simulink model "R7014E_QuadTankSim_IMC"  (R2025b)
settings: Solver=ode4  StartTime=0.0  StopTime=4000  FixedStep=0.01  RelTol=1e-3  EnableMultiTasking=on
values from neighbouring files (symbols this model uses):
  A1 = 28    [matlab_workspace.mat]
  a1 = 0.071    [matlab_workspace.mat]
  A2 = 32    [matlab_workspace.mat]
  a2 = 0.057    [matlab_workspace.mat]
  A3 = 28    [matlab_workspace.mat]
  a3 = 0.071    [matlab_workspace.mat]
  A4 = 32    [matlab_workspace.mat]
  a4 = 0.057    [matlab_workspace.mat]
  F_r_tilde_den = 1    [matlab_workspace.mat]
  F_r_tilde_num = 1    [matlab_workspace.mat]
  G11_den = [62.4182361958 1]    [matlab_workspace.mat]
  G11_num = [0 2.59815908165]    [matlab_workspace.mat]
  G22_den = [90.6440624664 1]    [matlab_workspace.mat]
  G22_num = [0 2.84679008684]    [matlab_workspace.mat]
  gamma1_M = 0.7    [matlab_workspace.mat]
  gamma2_M = 0.6    [matlab_workspace.mat]
  h1_init = 12.3    [matlab_workspace.mat]
  h2_init = 12.8    [matlab_workspace.mat]
  h3_init = 1.6    [matlab_workspace.mat]
  h4_init = 1.4    [matlab_workspace.mat]
  k1_M = 3.33    [matlab_workspace.mat]
  k2_M = 3.35    [matlab_workspace.mat]
  Q11_den = [23.3834317349 15.5889544899 2.59815908165]    [matlab_workspace.mat]
  Q11_num = [0 62.4182361958 1]    [matlab_workspace.mat]
  Q22_den = [25.6211107815 17.080740521 2.84679008684]    [matlab_workspace.mat]
  Q22_num = [0 90.6440624664 1]    [matlab_workspace.mat]
undefined symbols (not defined in the file or in its folder): sigbuilder_block
Description:
  | Double tank process simulation model
  | V1.0
  | 
  | Author: Wolfgang Birk, LTU
settings Model: MinMaxOverflowLogging=ForceOff  Creator=wolfgang  LastModifiedBy=kaspe
settings SolverCC: AlgebraicLoopSolver=TrustRegion
settings DataIOCC: LimitDataPoints=on  SaveFormat=Array  SignalLoggingSaveFormat=ModelDataLogs  ReturnWorkspaceOutputs=off
settings OptimizationCC: ExpressionDepthLimit=2147483647.0  LifeSpan=inf
settings DebuggingCC: UnderspecifiedInitializationDetection=Classic  MergeDetectMultiDrivingBlocksExec=none  SolverPrmCheckMsg=warning  FcnCallInpInsideContextMsg=warning  UnconnectedInputMsg=warning  UnconnectedOutputMsg=warning  UnconnectedLineMsg=warning  StateNameClashWarn=warning  SFUnexpectedBacktrackingDiag=warning  SFNoUnconditionalDefaultTransitionDiag=warning  SFExecutionAtInitializationDiag=none  ArithmeticOperatorsInVariantConditions=warning
settings HardwareCC: ProdBitPerPointer=32.0  ProdBitPerSizeT=32.0  ProdBitPerPtrDiffT=32.0  ProdLargestAtomicFloat=None  ProdIntDivRoundTo=Undefined  ProdEndianess=Unspecified  ProdWordSize=32.0  ProdHWDeviceType=32-bit Generic
settings ModelReferenceCC: EnableRefExpFcnMdlSchedulingChecks=on  PropagateSignalLabelsOutOfModel=off
settings SFSimCC: SimUseLocalCustomCode=off  CustomCodeUndefinedFunction=UseInterfaceOnly
settings RTWCC: RTWUseLocalCustomCode=off  GPUComputeCapability=3.5
settings CodeAppCC: StateflowObjectComments=on
settings GRTTargetCC: TargetLangStandard=C89/C90 (ANSI)
settings ConfigComp: CovMetricSettings=dw  CovSaveCumulativeToWorkspaceVar=on  CovSaveSingleToWorkspaceVar=on  CovExternalEMLEnable=off

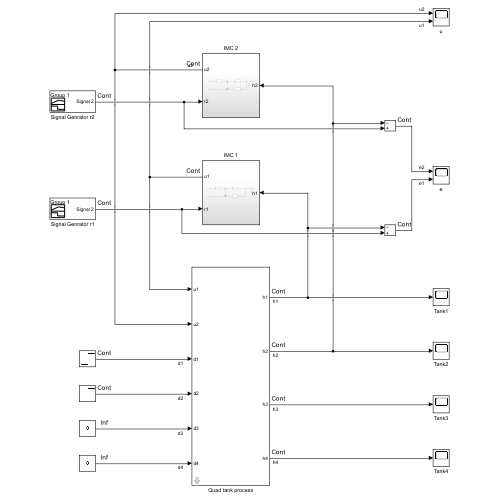
[thumbnail: Simulink's stored preview of the top-level diagram]
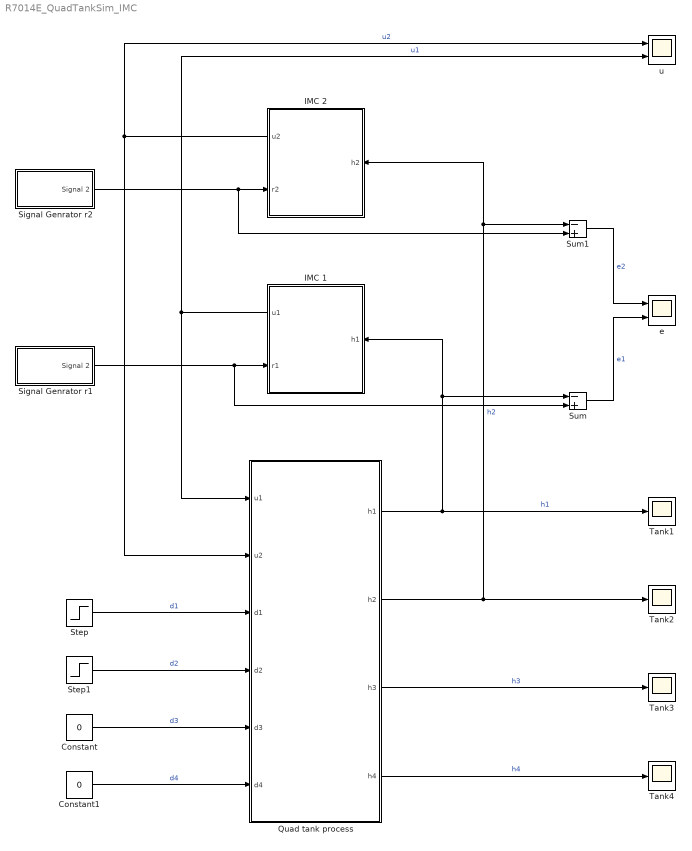
== system R7014E_QuadTankSim_IMC ==
  Constant : Constant  Value=0
  Constant1 : Constant  Value=0
  IMC 1 : Subsystem
      settings: PortSchema="{\"entries\":[{\"content\":{\"sides\":[{\"content\":{\"connectorIds\":[\"In1\"]},\"type\":\"ConnectorPlacement.EquallySpacedRectSide\",\"uuid\":\"4852cb48-3dbe-49d3-b52d-1f2b66e5782f\"},{\"content\":{\"connectorIds\":[\"Out1\",\"In2\"],\"side\":\"RIGHT\"},\"type\":\"ConnectorPlacement.EquallySpacedRectSide\",\"uuid\":\"9cc98c43-55ba-47ec-98d3-91ba0e651a74\"},{\"content\":{\"side\":\"TOP\"},\"type\":\"ConnectorPlacement.EquallySpacedRectSide\",\"uuid\":\"0e4ead2b-996b-4075-849e-a6886983cab4\"},{\"content\":{\"side\":\"BOTTOM\"},\"type\":\"ConnectorPlacement.EquallySpacedRectSide\",\"uuid\":\"443cd1da-2b11-4b7b-ba12-e267a6b444a4\"}]},\"type\":\"ConnectorPlacement.EquallySpacedConnector\",\"uuid\":\"d0829c27-0885-4d8f-a753-a80de6d2ea12\"}],\"packageUris\":[\"http://schema.mathworks.com/mf0/Connector/R2020b\"],\"version\":\"1.0\"}"
  IMC 2 : Subsystem
      settings: PortSchema="{\"entries\":[{\"content\":{\"sides\":[{\"content\":{\"connectorIds\":[\"In1\"]},\"type\":\"ConnectorPlacement.EquallySpacedRectSide\",\"uuid\":\"4852cb48-3dbe-49d3-b52d-1f2b66e5782f\"},{\"content\":{\"connectorIds\":[\"Out1\",\"In2\"],\"side\":\"RIGHT\"},\"type\":\"ConnectorPlacement.EquallySpacedRectSide\",\"uuid\":\"9cc98c43-55ba-47ec-98d3-91ba0e651a74\"},{\"content\":{\"side\":\"TOP\"},\"type\":\"ConnectorPlacement.EquallySpacedRectSide\",\"uuid\":\"0e4ead2b-996b-4075-849e-a6886983cab4\"},{\"content\":{\"side\":\"BOTTOM\"},\"type\":\"ConnectorPlacement.EquallySpacedRectSide\",\"uuid\":\"84a55638-02cd-431e-8938-8d2f80adb47b\"}]},\"type\":\"ConnectorPlacement.EquallySpacedConnector\",\"uuid\":\"d0829c27-0885-4d8f-a753-a80de6d2ea12\"}],\"packageUris\":[\"http://schema.mathworks.com/mf0/Connector/R2020b\"],\"version\":\"1.0\"}"
  Quad tank process : Subsystem  mask{hmax=20, A1=A1, ao1=a1, h10=h1_init, A2=A2, ao2=a2, h20=h2_init, A3=A3, ao3=a3, h30=h3_init, A4=A4, ao4=a4, h40=h4_init, k1=k1_M, k2=k2_M, gamma1=gamma1_M, gamma2=gamma2_M}
      mask prompts: hmax "Tank height (cm)"; A1 "Tank area (cm^2)"; ao1 "Opening area (cm^2)"; h10 "Initial level (cm)"; A2 "Tank area (cm^2)"; ao2 "Opening area (cm^2)"; h20 "Initial level (cm)"; A3 "Tank area (cm^2)"; ao3 "Opening area (cm^2)"; h30 "Initial level (cm)"; A4 "Tank area (cm^2)"; ao4 "Opening area (cm^2)"; h40 "Initial level (cm)"; k1 "Pump1 gain (cm^3/V/s)"; k2 "Pump2 gain (cm^3/V/s)"; gamma1 "Split valve gamma 1"; gamma2 "Split valve gamma 2"
      mask help: Double tank process parameters
      mask DialogControl Container3 Prompt: General parameters
      mask DialogControl ParameterGroupVar Prompt: Tank 1
      mask DialogControl ParameterGroupVar_copy_copy_copy Prompt: Tank 2
      mask DialogControl ParameterGroupVar_copy_copy Prompt: Tank 3
      mask DialogControl ParameterGroupVar_copy Prompt: Tank 4
      mask DialogControl Container4 Prompt: Pump parameters
  Signal Genrator r1 : Subsystem  Tag=STV Subsys  LoadFcn=sigbuilder_block('load');  StartFcn=sigbuilder_block('start');  StopFcn=sigbuilder_block('stop');  ClipboardFcn=sigbuilder_block('clipboard');  mask(Sigbuilder block){tuvar=[0:10]}
      mask help: Simulink:masks:SigbuilderBlock_MD
      mask init:
      | if ~strcmp(get_param(bdroot(gcbh),'SimulationStatus'),'stopped') tuvar = sigbuilder_block('maskInit'); end
      settings: CopyFcn=sigbuilder_block('copy');  DeleteFcn=sigbuilder_block('delete');  ModelCloseFcn=sigbuilder_block('modelClose');  PreSaveFcn=sigbuilder_block('preSave');  PauseFcn=sigbuilder_block('pause');  ContinueFcn=sigbuilder_block('continue');  NameChangeFcn=sigbuilder_block('namechange');  OpenFcn=sigbuilder_block('open',[289.5 231.75 954.75 575.25 ]);  CloseFcn=sigbuilder_block('close');
      mask Display: plot(0, 0, 100, 100,[2, 2, 32, 32, 2], [68, 8, 8, 68, 68],[32, 2], [38, 38], [32, 19, 2],[53, 60, 44], [32, 17, 17, 2],[16, 16, 31, 31]);txt = getActiveGroup(gcbh);text(2, 100, txt,'verticalAlignment', 'top');
  Signal Genrator r2 : Subsystem  Tag=STV Subsys  LoadFcn=sigbuilder_block('load');  StartFcn=sigbuilder_block('start');  StopFcn=sigbuilder_block('stop');  ClipboardFcn=sigbuilder_block('clipboard');  mask(Sigbuilder block){tuvar=[0:10]}
      mask help: Simulink:masks:SigbuilderBlock_MD
      mask init:
      | if ~strcmp(get_param(bdroot(gcbh),'SimulationStatus'),'stopped') tuvar = sigbuilder_block('maskInit'); end
      settings: CopyFcn=sigbuilder_block('copy');  DeleteFcn=sigbuilder_block('delete');  ModelCloseFcn=sigbuilder_block('modelClose');  PreSaveFcn=sigbuilder_block('preSave');  PauseFcn=sigbuilder_block('pause');  ContinueFcn=sigbuilder_block('continue');  NameChangeFcn=sigbuilder_block('namechange');  OpenFcn=sigbuilder_block('open',[289.5 231.75 954.75 575.25 ]);  CloseFcn=sigbuilder_block('close');
      mask Display: plot(0, 0, 100, 100,[2, 2, 32, 32, 2], [68, 8, 8, 68, 68],[32, 2], [38, 38], [32, 19, 2],[53, 60, 44], [32, 17, 17, 2],[16, 16, 31, 31]);txt = getActiveGroup(gcbh);text(2, 100, txt,'verticalAlignment', 'top');
  Step : Step  Time=1500  After=0.25  SampleTime=0
  Step1 : Step  Time=2700  After=0.25  SampleTime=0
  Sum : Sum  Inputs=-+
  Sum1 : Sum  Inputs=-+
  Tank{1..4} (4 alike) : Scope
      Tank1 settings: TimeSpan=100  ActiveDisplayYMinimum=11.085608549570658  ActiveDisplayYMaximum=15.73381463003302
      Tank2 settings: TimeSpan=100  ActiveDisplayYMinimum=14.432025090540726  ActiveDisplayYMaximum=14.874075426686041  DataLoggingVariableName=ScopeData3
      Tank3 settings: TimeSpan=100  ActiveDisplayYMinimum=1.57505  ActiveDisplayYMaximum=1.66866
      Tank4 settings: TimeSpan=100  ActiveDisplayYMinimum=1.35987  ActiveDisplayYMaximum=1.45363  DataLoggingVariableName=ScopeData2
  e : Scope  NumInputPorts=2
      settings: TimeSpan=100  ActiveDisplayYMinimum=-0.42634096919183645  ActiveDisplayYMaximum=2.269870155777078  DataLoggingVariableName=ScopeData5
  u : Scope  NumInputPorts=2
      settings: TimeSpan=100  ActiveDisplayYMinimum=-1.213965917934767  ActiveDisplayYMaximum=10.925693261412906  DataLoggingVariableName=ScopeData4
  wires:
  Quad tank process/3(h3) -> Tank3/1  "h3"
  Quad tank process/1(h1) -> IMC 1/1(h1), Sum/1, Tank1/1  "h1"
  Step/1 -> Quad tank process/3(d1)  "d1"
  Step1/1 -> Quad tank process/4(d2)  "d2"
  Constant/1 -> Quad tank process/5(d3)  "d3"
  Constant1/1 -> Quad tank process/6(d4)  "d4"
  Quad tank process/2(h2) -> Tank2/1, IMC 2/1(h2), Sum1/1  "h2"
  Quad tank process/4(h4) -> Tank4/1  "h4"
  IMC 1/1(u1) -> u/2, Quad tank process/1(u1)  "u1"
  Signal Genrator r1/1(Signal 2) -> IMC 1/2(r1), Sum/2
  Signal Genrator r2/1(Signal 2) -> IMC 2/2(r2), Sum1/2
  IMC 2/1(u2) -> u/1, Quad tank process/2(u2)  "u2"
  Sum1/1 -> e/1  "e2"
  Sum/1 -> e/2  "e1"

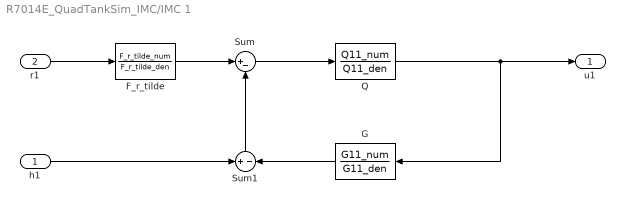
== system R7014E_QuadTankSim_IMC/IMC 1 ==
  h1 : Inport
  r1 : Inport  Port=2
  F_r_tilde : TransferFcn  Numerator=F_r_tilde_num  Denominator=F_r_tilde_den
  G : TransferFcn  Numerator=G11_num  Denominator=G11_den
  Q : TransferFcn  Numerator=Q11_num  Denominator=Q11_den
  Sum : Sum  Inputs=|+-
  Sum1 : Sum  Inputs=+|-
  u1 : Outport
  wires:
  F_r_tilde/1 -> Sum/1
  r1/1 -> F_r_tilde/1
  Sum/1 -> Q/1
  Sum1/1 -> Sum/2
  Q/1 -> G/1, u1/1
  G/1 -> Sum1/2
  h1/1 -> Sum1/1

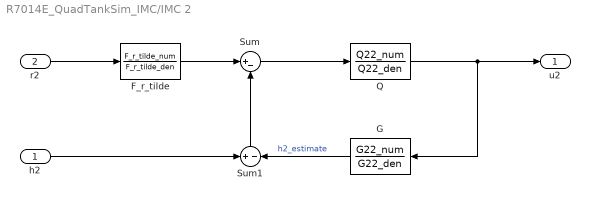
== system R7014E_QuadTankSim_IMC/IMC 2 ==
  h2 : Inport
  r2 : Inport  Port=2
  F_r_tilde : TransferFcn  Numerator=F_r_tilde_num  Denominator=F_r_tilde_den
  G : TransferFcn  Numerator=G22_num  Denominator=G22_den
  Q : TransferFcn  Numerator=Q22_num  Denominator=Q22_den
  Sum : Sum  Inputs=|+-
  Sum1 : Sum  Inputs=+|-
  u2 : Outport
  wires:
  F_r_tilde/1 -> Sum/1
  r2/1 -> F_r_tilde/1
  Sum/1 -> Q/1
  Sum1/1 -> Sum/2
  Q/1 -> u2/1, G/1
  h2/1 -> Sum1/1
  G/1 -> Sum1/2  "h2_estimate"

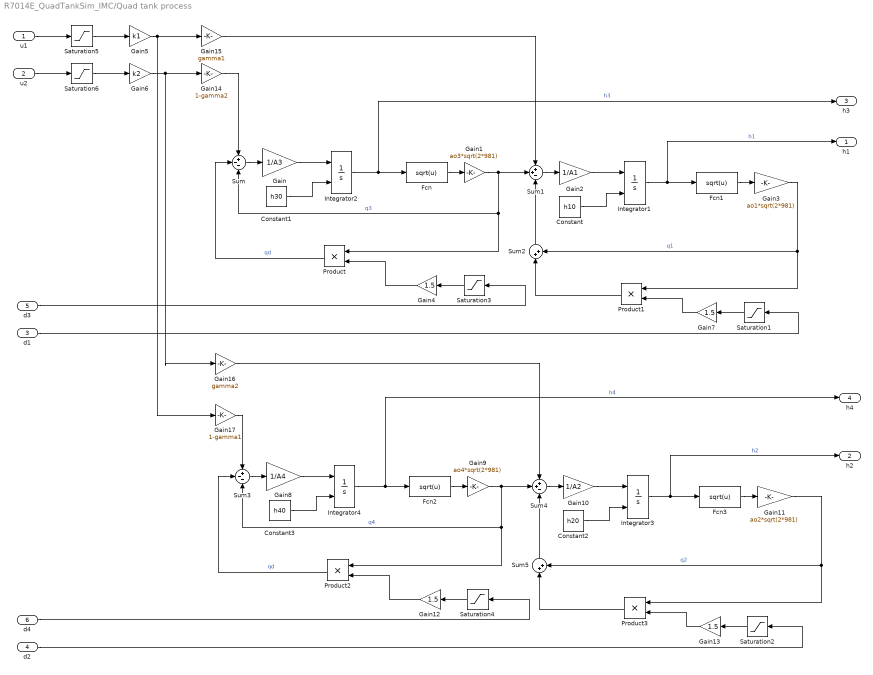
== system R7014E_QuadTankSim_IMC/Quad tank process ==
  u1 : Inport
  u2 : Inport  Port=2
  d1 : Inport  Port=3
  d2 : Inport  Port=4
  d3 : Inport  Port=5
  d4 : Inport  Port=6
  Constant : Constant  Value=h10
  Constant1 : Constant  Value=h30
  Constant2 : Constant  Value=h20
  Constant3 : Constant  Value=h40
  Fcn{,1..3} (4 alike) : Fcn  Expr=sqrt(u)
  Gain : Gain  Gain=1/A3
  Gain1 : Gain  Gain=ao3*sqrt(2*981)
  Gain10 : Gain  Gain=1/A2
  Gain11 : Gain  Gain=ao2*sqrt(2*981)
  Gain{4,7,12..13} (4 alike) : Gain  Gain=1.5
  Gain14 : Gain  Gain=1-gamma2
  Gain15 : Gain  Gain=gamma1
  Gain16 : Gain  Gain=gamma2
  Gain17 : Gain  Gain=1-gamma1
  Gain2 : Gain  Gain=1/A1
  Gain3 : Gain  Gain=ao1*sqrt(2*981)
  Gain5 : Gain  Gain=k1
  Gain6 : Gain  Gain=k2
  Gain8 : Gain  Gain=1/A4
  Gain9 : Gain  Gain=ao4*sqrt(2*981)
  Integrator{1..4} (4 alike) : Integrator  InitialConditionSource=external  LimitOutput=on  UpperSaturationLimit=hmax  LowerSaturationLimit=0
  Product{,1..3} (4 alike) : Product  RndMeth=Zero
  Saturation{1..4} (4 alike) : Saturate  UpperLimit=1  LowerLimit=0
  Saturation5 : Saturate  UpperLimit=10  LowerLimit=0
  Saturation6 : Saturate  UpperLimit=10  LowerLimit=0
  Sum : Sum  Inputs=+--
  Sum1 : Sum  Inputs=++-
  Sum2 : Sum  Inputs=|++
  Sum3 : Sum  Inputs=+--
  Sum4 : Sum  Inputs=++-
  Sum5 : Sum  Inputs=|++
  h1 : Outport  VectorParamsAs1DForOutWhenUnconnected=off
  h2 : Outport  Port=2  VectorParamsAs1DForOutWhenUnconnected=off
  h3 : Outport  Port=3  VectorParamsAs1DForOutWhenUnconnected=off
  h4 : Outport  Port=4  VectorParamsAs1DForOutWhenUnconnected=off
  wires:
  Sum/1 -> Gain/1
  Gain/1 -> Integrator2/1
  Fcn/1 -> Gain1/1
  Gain1/1 -> Product/1, Sum/3, Sum1/2  "q3"
  Sum1/1 -> Gain2/1
  Gain2/1 -> Integrator1/1
  Fcn1/1 -> Gain3/1
  Integrator2/1 -> h3/1, Fcn/1  "h3"
  Product/1 -> Sum/2  "qd"
  d3/1 -> Saturation3/1
  Integrator1/1 -> h1/1, Fcn1/1  "h1"
  Saturation3/1 -> Gain4/1
  Gain4/1 -> Product/2
  u1/1 -> Saturation5/1
  Constant/1 -> Integrator1/2
  Constant1/1 -> Integrator2/2
  u2/1 -> Saturation6/1
  Gain5/1 -> Gain17/1, Gain15/1
  Sum2/1 -> Sum1/3
  Gain3/1 -> Product1/1, Sum2/2  "q1"
  Gain7/1 -> Product1/2
  Saturation1/1 -> Gain7/1
  d1/1 -> Saturation1/1
  Product1/1 -> Sum2/1
  Product3/1 -> Sum5/1
  d2/1 -> Saturation2/1
  Saturation2/1 -> Gain13/1
  Gain13/1 -> Product3/2
  Gain11/1 -> Sum5/2, Product3/1  "q2"
  Sum5/1 -> Sum4/3
  Constant3/1 -> Integrator4/2
  Constant2/1 -> Integrator3/2
  Gain12/1 -> Product2/2
  Saturation4/1 -> Gain12/1
  Integrator3/1 -> Fcn3/1, h2/1  "h2"
  d4/1 -> Saturation4/1
  Product2/1 -> Sum3/2  "qd"
  Integrator4/1 -> h4/1, Fcn2/1  "h4"
  Fcn3/1 -> Gain11/1
  Gain10/1 -> Integrator3/1
  Sum4/1 -> Gain10/1
  Gain9/1 -> Sum4/2, Sum3/3, Product2/1  "q4"
  Fcn2/1 -> Gain9/1
  Gain8/1 -> Integrator4/1
  Sum3/1 -> Gain8/1
  Gain14/1 -> Sum/1
  Gain15/1 -> Sum1/1
  Gain6/1 -> Gain16/1, Gain14/1
  Gain16/1 -> Sum4/1
  Gain17/1 -> Sum3/1
  Saturation5/1 -> Gain5/1
  Saturation6/1 -> Gain6/1

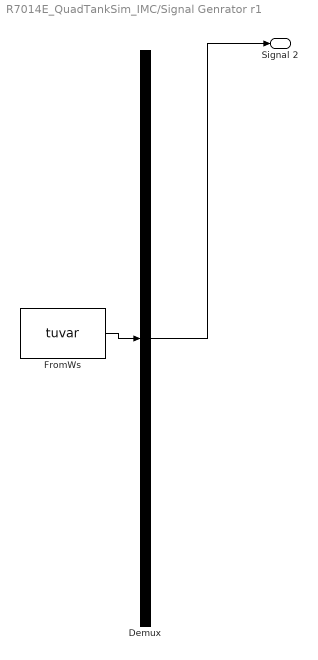
== system R7014E_QuadTankSim_IMC/Signal Genrator r1 ==
  Demux : Demux  Tag=STV Demux  Outputs=1
      settings: DisplayOption=none
  FromWs : FromWorkspace  Tag=STV FromWs  VariableName=tuvar
      SigBuilderData=|
      | common.afterFinalStr = 'Extrapolate'
      | common.sampleTime = 0
      | dataSet.timeRange = [0 2000]
      | dataSet.name = 'Group 1'
      | sbobj.Groups.Name = 'Group 1'
      | sbobj.Groups.Signals.Name = 'Signal 2'
      | sbobj.Groups.Signals.XData = [0 500 500 2000]
      | sbobj.Groups.Signals.YData = [12.3 12.3 14.3 14.3]
      | sbobj.Groups.TimeRange = [0 2000]
  Signal 2 : Outport  Tag=STV Outport
  wires:
  FromWs/1 -> Demux/1
  Demux/1 -> Signal 2/1

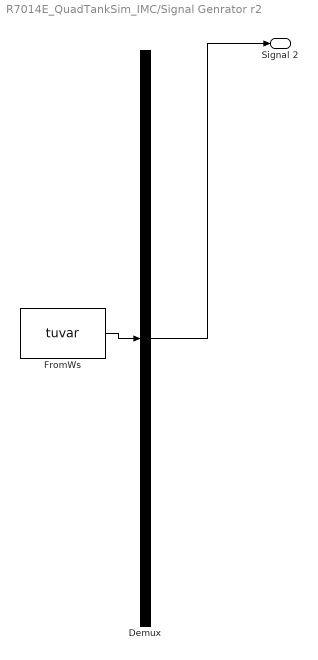
== system R7014E_QuadTankSim_IMC/Signal Genrator r2 ==
  Demux : Demux  Tag=STV Demux  Outputs=1
      settings: DisplayOption=none
  FromWs : FromWorkspace  Tag=STV FromWs  VariableName=tuvar
      SigBuilderData=|
      | common.afterFinalStr = 'Extrapolate'
      | common.sampleTime = 0
      | dataSet.timeRange = [0 2000]
      | dataSet.name = 'Group 1'
      | sbobj.Groups.Name = 'Group 1'
      | sbobj.Groups.Signals.Name = 'Signal 2'
      | sbobj.Groups.Signals.XData = [0 1000 1000 2000]
      | sbobj.Groups.Signals.YData = [12.8 12.8 14.8 14.8]
      | sbobj.Groups.TimeRange = [0 2000]
  Signal 2 : Outport  Tag=STV Outport
  wires:
  FromWs/1 -> Demux/1
  Demux/1 -> Signal 2/1
